simulink model "MRACSBR"  (R2022b)
settings: Solver=FixedStepAuto  StartTime=0.0  StopTime=inf  FixedStep=0.01  RelTol=1e-3
libraries: arduinolib x2, arduinosensorlib x1
settings Model: SimulationMode=external  ExtModeTrigDuration=2  Creator=edgar  LastModifiedBy=laksh
settings SolverCC: AllowMultiTaskInputOutput=on  AutoInsertRateTranBlk=on
settings OptimizationCC: EnhancedBackFolding=on  PassReuseOutputArgsAs=Individual arguments  ZeroExternalMemoryAtStartup=off  ZeroInternalMemoryAtStartup=off  MaxStackSize=64  OptimizeBlockOrder=speed  DifferentSizesBufferReuse=on  OptimizationCustomize=off  EfficientTunableParamExpr=on
settings DebuggingCC: ParameterTunabilityLossMsg=error
settings HardwareCC: ProdBitPerInt=16  ProdBitPerPointer=16  ProdBitPerSizeT=16  ProdBitPerPtrDiffT=16  ProdLargestAtomicFloat=None  ProdWordSize=8  ProdLongLongMode=on  ProdHWDeviceType=Atmel->AVR  UseEmbeddedCoderFeatures=off  UseSimulinkCoderFeatures=off
settings ModelReferenceCC: EnableRefExpFcnMdlSchedulingChecks=on
settings SFSimCC: MATLABDynamicMemAlloc=off
settings RTWCC: Description=Embedded Coder  SystemTargetFile=ert.tlc  HardwareBoard=Arduino Uno  TemplateMakefile=ert_default_tmf  RTWVerbose=off  Toolchain=Arduino AVR  BuildConfiguration=Faster Runs
settings CodeAppCC: ForceParamTrailComments=on  OperatorAnnotations=on  SimulinkDataObjDesc=on  SFDataObjDesc=on  MangleLength=10  InsertBlockDesc=on
settings ERTTargetCC: SupportContinuousTime=on  SupportNonInlinedSFcns=on  SupportVariableSizeSignals=on  ExtMode=on  ExtModeTransport=3  ExtModeStaticAlloc=on  ExtModeAutomaticAllocSize=off  ExtModeStaticAllocSize=250  ExtModeMexFile=ext_xcp  ExtModeMexArgs=0 11 115200  ExtModeIntrfLevel=Level2 - Open  ERTSrcFileBannerTemplate=codertarget_code_template.cgt  ERTHdrFileBannerTemplate=codertarget_code_template.cgt  ERTDataSrcFileTemplate=codertarget_code_template.cgt  ERTDataHdrFileTemplate=codertarget_code_template.cgt

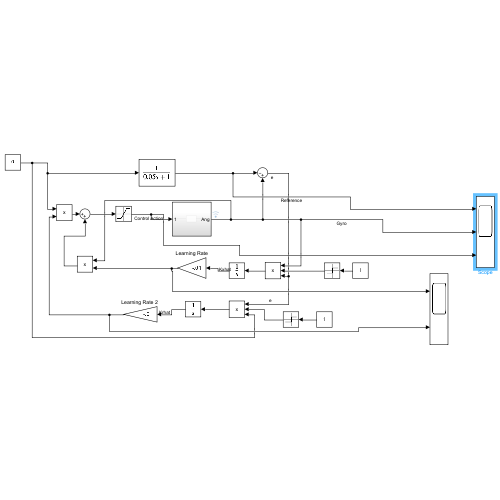
[thumbnail: Simulink's stored preview of the top-level diagram]
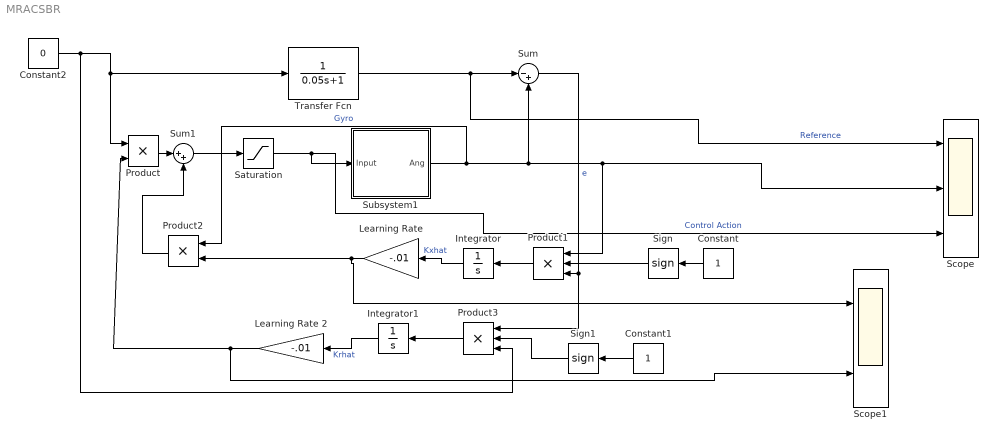
== system MRACSBR ==
  Constant : Constant
  Constant1 : Constant
  Constant2 : Constant  Value=0
  Integrator : Integrator  InitialCondition=-15  UpperSaturationLimit=1000  LowerSaturationLimit=-1000
  Integrator1 : Integrator  InitialCondition=15  UpperSaturationLimit=1000  LowerSaturationLimit=-1000  AbsoluteTolerance=-1
  Learning Rate : Gain  Gain=-.01
  "Learning Rate 2 " : Gain  Gain=-.01
  Product : Product
  Product1 : Product  Inputs=3
  Product2 : Product
  Product3 : Product  Inputs=3
  Saturation : Saturate  UpperLimit=180  LowerLimit=-180
  Scope : Scope  NumInputPorts=3
  Scope1 : Scope  NumInputPorts=2
  Sign : Signum
  Sign1 : Signum
  Subsystem1 : Subsystem
  Sum : Sum  Inputs=|-+
  Sum1 : Sum  Inputs=|++
  Transfer Fcn : TransferFcn  Denominator=[0.05 1]
  wires:
  Sum1/1 -> Saturation/1
  Product/1 -> Sum1/1
  Constant/1 -> Sign/1
  Product1/1 -> Integrator/1
  Integrator/1 -> Learning Rate/1  "Kxhat"
  Constant1/1 -> Sign1/1
  Integrator1/1 -> "Learning Rate 2 "/1  "Krhat"
  Product3/1 -> Integrator1/1
  Product2/1 -> Sum1/2
  Sign/1 -> Product1/2
  Sum/1 -> Product3/1, Product1/3  "e"
  Sign1/1 -> Product3/2
  Saturation/1 -> Subsystem1/1(Input), Scope/3  "Control Action"
  Subsystem1/1(Ang) -> Product2/1, Sum/2, Product1/1, Scope/2  "Gyro"
  Transfer Fcn/1 -> Scope/1, Sum/1  "Reference"
  Constant2/1 -> Product3/3, Product/1, Transfer Fcn/1
  Learning Rate/1 -> Scope1/1, Product2/2
  "Learning Rate 2 "/1 -> Product/2, Scope1/2

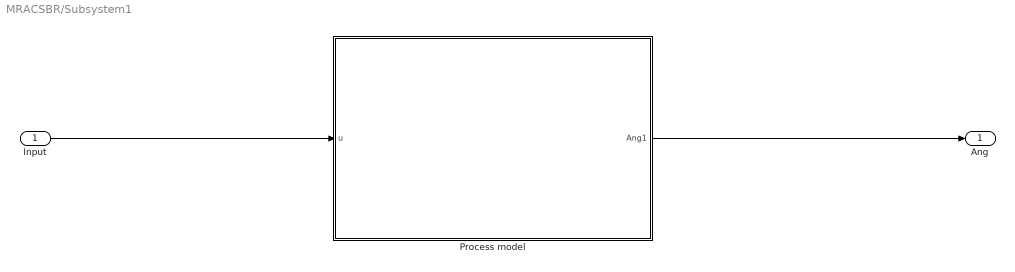
== system MRACSBR/Subsystem1 ==
  Input : Inport
  Process model : Subsystem
  Ang : Outport
  wires:
  Process model/1(Ang1) -> Ang/1
  Input/1 -> Process model/1(u)

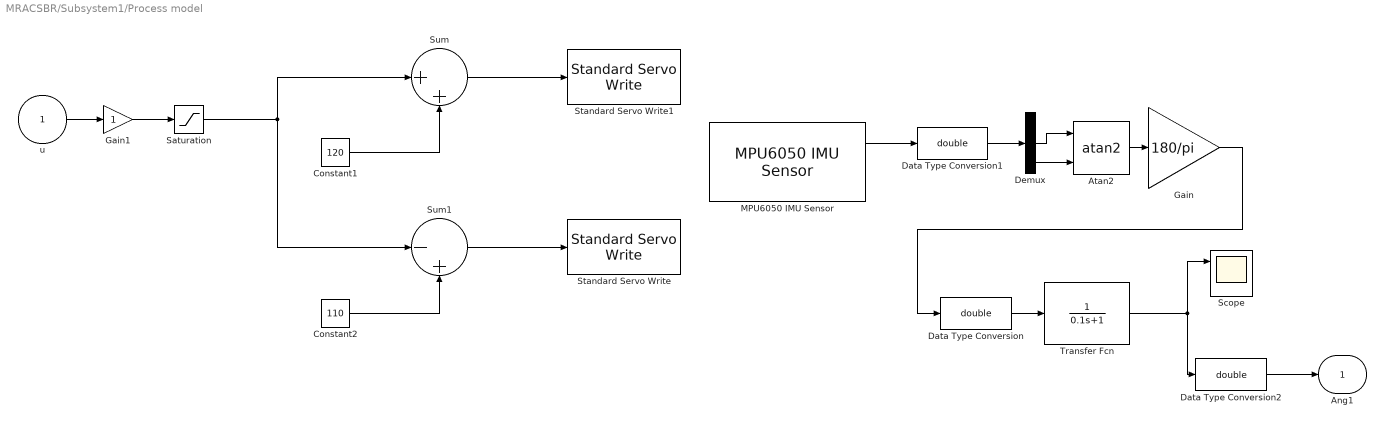
== system MRACSBR/Subsystem1/Process model ==
  u : Inport
  Atan2 : Trigonometry  Operator=atan2
  Constant1 : Constant  Value=120
  Constant2 : Constant  Value=110
  Data Type Conversion : DataTypeConversion  OutDataTypeStr=double  SaturateOnIntegerOverflow=off  RndMeth=Floor
  Data Type Conversion1 : DataTypeConversion  OutDataTypeStr=double  SaturateOnIntegerOverflow=off  RndMeth=Floor
  Data Type Conversion2 : DataTypeConversion  OutDataTypeStr=double  SaturateOnIntegerOverflow=off  RndMeth=Floor
  Demux : Demux  Outputs=3
  Gain : Gain  Gain=180/pi
  Gain1 : Gain
  MPU6050 IMU Sensor : arduinosensorlib/MPU6050 IMU Sensor  SlaveAddress=0x68  Accel=on  AngularRate=on  Temperature=off  Status=off  Timestamp=off  EulerAngles=off  Quat=off  AccelRange=4G  GyroRange=500 dps  DmpOdr=200 Hz  Dlpf=Accelerometer: 184Hz, Gyroscope: 188Hz  spf=1  SampleTime=-1  QueueSizeFactor=1
  Saturation : Saturate  UpperLimit=180  LowerLimit=-180
  Scope : Scope  NumInputPorts=2
  Standard Servo Write : arduinolib/Standard Servo Write  pinNumber=3  ServoIndex=0  blockPlatform=ARDUINO
  Standard Servo Write1 : arduinolib/Standard Servo Write  pinNumber=6  ServoIndex=1  blockPlatform=ARDUINO
  Sum : Sum  Inputs=|++
  Sum1 : Sum  Inputs=|-+
  Transfer Fcn : TransferFcn  Denominator=[0.1 1]
  Ang1 : Outport
  wires:
  MPU6050 IMU Sensor/1 -> Data Type Conversion1/1
  Data Type Conversion1/1 -> Demux/1
  Constant1/1 -> Sum/2
  Sum/1 -> Standard Servo Write1/1
  Sum1/1 -> Standard Servo Write/1
  Demux/2 -> Atan2/1
  Constant2/1 -> Sum1/2
  Demux/3 -> Atan2/2
  Atan2/1 -> Gain/1
  u/1 -> Gain1/1
  Gain/1 -> Data Type Conversion/1
  Transfer Fcn/1 -> Data Type Conversion2/1, Scope/1
  Data Type Conversion/1 -> Transfer Fcn/1
  Saturation/1 -> Sum1/1, Sum/1
  Gain1/1 -> Saturation/1
  Data Type Conversion2/1 -> Ang1/1
